simulink model "Ej_01"  (R2020a)
settings: Solver=VariableStepAuto  StartTime=0.0  StopTime=10  RelTol=1e-3
libraries: roblocks x6
settings Model: Creator=Owner  LastModifiedBy=sebas
settings DataIOCC: ReturnWorkspaceOutputs=off
settings DebuggingCC: ArithmeticOperatorsInVariantConditions=warning
settings SFSimCC: SimUseLocalCustomCode=off  CustomCodeUndefinedFunction=UseInterfaceOnly
settings RTWCC: RTWUseLocalCustomCode=off

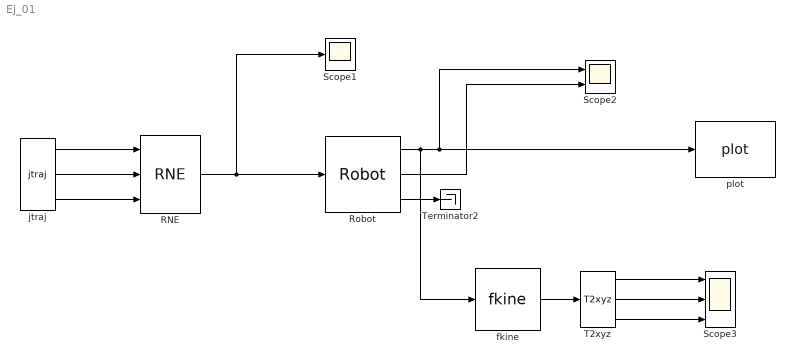
== system Ej_01 ==
  RNE : roblocks/Arm/RNE  robot=messi  grav=[0 0 9.81]
  Robot : roblocks/Arm/Robot  robot=messi  q0=[-pi/2 pi/2]
  Scope1 : Scope
  Scope2 : Scope  NumInputPorts=2
  Scope3 : Scope  NumInputPorts=3
  T2xyz : roblocks/Toolbox/T2xyz
  Terminator2 : Terminator
  fkine : roblocks/Arm/fkine  robot=messi
  jtraj : roblocks/Toolbox/jtraj  q0=q1  qf=q2  tmax=10  ts=-1
  plot : roblocks/Arm/plot  robot=messi  fps=5  holdplot=on
  wires:
  jtraj/1 -> RNE/1
  jtraj/2 -> RNE/2
  jtraj/3 -> RNE/3
  RNE/1 -> Scope1/1, Robot/1
  Robot/1 -> fkine/1, Scope2/1, plot/1
  Robot/3 -> Terminator2/1
  Robot/2 -> Scope2/2
  fkine/1 -> T2xyz/1
  T2xyz/1 -> Scope3/1
  T2xyz/2 -> Scope3/2
  T2xyz/3 -> Scope3/3
